simulink model "fwv_2020b"  (R2020b)
settings: Solver=ode15s  StartTime=0.0  StopTime=1  RelTol=1e-3  AbsTol=1e-3  EnableMultiTasking=on
model workspace: external: MATLAB File /home/jeff/文档/research/fwvlab/main.m (data not in the file)
values from neighbouring files (symbols this model uses):
  A_D = 1.5    [main.m]    (also in param.m; params.m)
  A_L = 1.8    [main.m]    (also in param.m; params.m)
  c_bar = S/R    (= 0.0357142857143)    [main.m]    (also in param.m = 0.0251327412287; params.m)
  C_D0 = 0.45    [main.m]    (also in param.m; params.m)
  m = 2    [rbf_pid.m]
  r00 = double(int(f,[0,1]))    [main.m]    (also in param.m = 1; params.m = 0.933333333333)
  r11 = double(int(x*f,[0,1]))    [main.m]    (also in param.m = double(int(curv(x)*(x+1/9),0,1)); params.m = 0.481185185185)
  r22 = double(int(x^2*f,[0,1]))    [main.m]    (also in param.m = double(int(curv(x)*(x+1/9)^2,0,1)); params.m = 0.304750617284)
  r33 = double(int(x^3*f,[0,1]))    [main.m]    (also in param.m = double(int(curv(x)*(x+1/9)^3,0,1)); params.m = 0.218568691358)
  r_cp = Rw*r33/r22    [main.m]    (also in param.m; params.m = 0.10758076225)
  rho = 1.205    [main.m]    (also in param.m; params.m)
  Rw = 0.15    [main.m]    (also in param.m = 0.075; params.m)
  z0 = double(int(f^2,[0,1]))    [main.m]
  z1 = double(int(x*f^2,[0,1]))    [main.m]
  z2 = double(int(x^2*f^2,[0,1]))    [main.m]
undefined symbols (not defined in the file or in its folder): X, Y, Z
libraries: sm_lib x45, nesl_utility x38
(part 2 of 2)

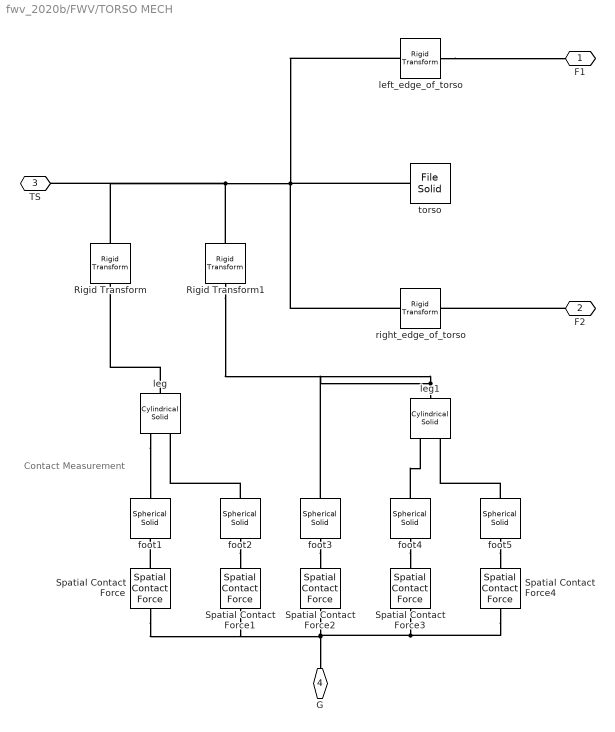
== system fwv_2020b/FWV/TORSO MECH ==
  note: Contact Measurement
  Rigid Transform : sm_lib/Frames and Transforms/Rigid Transform  TranslationMethod=StandardAxis  TranslationStandardOffset=6.25  TranslationLengthUnit=cm  TranslationStandardAxis=-Z  TranslationCartesianOffset=[0 0 0]  TranslationROffset=0  TranslationROffsetUnits=m  TranslationZOffset=0  TranslationZOffsetUnits=m  TranslationThetaOffset=0  TranslationThetaOffsetUnits=deg  RotationMethod=RotationSequence  RotationAngleUnits=deg  RotationStandardAxis=+Y  RotationAngle=90  RotationArbitraryAxis=[0 0 1]  FollAlignAxisA=+X  BaseAlignAxisA=+Y  FollAlignAxisB=+Y  BaseAlignAxisB=+Z  RotationSequenceAxes=FollowerAxes  RotationSequence=ZYX  RotationSequenceAngles=[45 90 0]  RotationSequenceAnglesUnits=deg  RotationMatrix=[1 0 0; 0 1 0; 0 0 1]
  Rigid Transform1 : sm_lib/Frames and Transforms/Rigid Transform  TranslationMethod=StandardAxis  TranslationStandardOffset=6.25  TranslationLengthUnit=cm  TranslationStandardAxis=-Z  TranslationCartesianOffset=[0 0 0]  TranslationROffset=0  TranslationROffsetUnits=m  TranslationZOffset=0  TranslationZOffsetUnits=m  TranslationThetaOffset=0  TranslationThetaOffsetUnits=deg  RotationMethod=RotationSequence  RotationAngleUnits=deg  RotationStandardAxis=+X  RotationAngle=90  RotationArbitraryAxis=[0 0 1]  FollAlignAxisA=+X  BaseAlignAxisA=+Y  FollAlignAxisB=+Y  BaseAlignAxisB=+Z  RotationSequenceAxes=FollowerAxes  RotationSequence=ZYX  RotationSequenceAngles=[-45 90 0]  RotationSequenceAnglesUnits=deg  RotationMatrix=[1 0 0; 0 1 0; 0 0 1]
  Spatial Contact Force{,1..4} (5 alike) : sm_lib/Forces and Torques/Spatial Contact Force  CoefficientOfDynamicFriction=mu1  CoefficientOfStaticFriction=mu0  SenseContactBaseRotation=off  SenseContactBaseTranslation=off  NormalDamping=1e3  NormalDampingUnits=N/(m/s)  SenseContactFollowerRotation=off  SenseContactFollowerTranslation=off  SenseContactSignal=off  NormalStiffness=1e6  NormalStiffnessUnits=N/m  FrictionalCriticalVelocity=1e-3  FrictionalCriticalVelocityUnits=m/s  ZeroCrossDetectContactStartAndEnd=off  FrictionType=SmoothStickSlip  SenseFrictionalForceMagnitude=off  SenseNormalForceMagnitude=off  NormalForceType=SmoothSpringDamper  SenseNormalVelocity=off  SenseSeparationDistance=off  SenseTangentialVelocity=off  SenseTangentialVelocityMagnitude=off  NormalTransitionRegionWidth=1e-4  NormalTransitionRegionWidthUnits=m
  foot{1..5} (5 alike) : sm_lib/Body Elements/Spherical Solid  GraphicAmbientColor=[0.15 0.15 0.15 1.0]  BasedOnType=Density  CenterOfMass=[0 0 0]  CenterOfMassUnits=m  GraphicDiffuseColor=[0.5 0.5 0.5]  Density=1000  DensityUnits=kg/m^3  DoExposeReferenceFrame=on  GraphicEmissiveColor=[0.0 0.0 0.0 1.0]  ExportEntireGeometry=on  SerializedExposedGeometries=<ExposedGeometries><ExposedGeometry><RawGeometryId>entire</RawGeometryId><ExposedGeometryId>G</ExposedGeometryId></ExposedGeometry></ExposedGeometries>  SerializedFrames=<Frames/>  MarkerShape=Sphere  MarkerSize=10  GraphicType=FromGeometry  InertiaType=Custom  Mass=0  MassUnits=kg  MomentsOfInertia=[1 1 1]  MomentsOfInertiaUnits=kg*m^2  GraphicOpacity=1.0  ProductsOfInertia=[0 0 0]  ProductsOfInertiaUnits=kg*m^2  GraphicShininess=75  GraphicSpecularColor=[0.5 0.5 0.5 1.0]  SphereRadius=0.25  SphereRadiusUnits=cm  GraphicVisPropType=SimpleVisualProperties
  left_edge_of_torso : sm_lib/Frames and Transforms/Rigid Transform  TranslationMethod=Cartesian  TranslationStandardOffset=0  TranslationLengthUnit=cm  TranslationStandardAxis=+Z  TranslationCartesianOffset=[0 4 0]  TranslationROffset=0  TranslationROffsetUnits=m  TranslationZOffset=0  TranslationZOffsetUnits=m  TranslationThetaOffset=0  TranslationThetaOffsetUnits=deg  RotationMethod=None  RotationAngleUnits=deg  RotationStandardAxis=+Z  RotationAngle=0.0  RotationArbitraryAxis=[0 0 1]  FollAlignAxisA=+X  BaseAlignAxisA=+Y  FollAlignAxisB=+Y  BaseAlignAxisB=+Z  RotationSequenceAxes=FollowerAxes  RotationSequence=XYX  RotationSequenceAngles=[0 0 0]  RotationSequenceAnglesUnits=deg  RotationMatrix=[1 0 0; 0 1 0; 0 0 1]
  leg : sm_lib/Body Elements/Cylindrical Solid  GraphicAmbientColor=[0.15 0.15 0.15 1.0]  BasedOnType=Density  CenterOfMass=[0 0 0]  CenterOfMassUnits=m  GraphicDiffuseColor=[0.5 0.5 0.5]  CylinderLength=160  CylinderLengthUnits=mm  CylinderRadius=2.5  CylinderRadiusUnits=mm  Density=1000  DensityUnits=kg/m^3  DoExposeReferenceFrame=on  GraphicEmissiveColor=[0.0 0.0 0.0 1.0]  ExportEntireGeometry=off  SerializedFrames=<Frames><Frame><Id>Frame1</Id><Value><Name>F1</Name><Origin><Source>GeometricFeature</Source><FeatureName>top curve</FeatureName></Origin><PrimaryAxis><DefinedDirection>+Z</DefinedDirection><Source>ReferenceFrame</Source><SourceDirection>+Z</SourceDirection><FeatureName></FeatureName></PrimaryAxis><SecondaryAxis><DefinedDirection>+X</DefinedDirection><Source>ReferenceFrame</Source><SourceDirection>+X</SourceDirection><FeatureName></FeatureName></SecondaryAxis></Value></Frame><Frame><Id>Frame2</Id><Value><Name>F2</Name><Origin><Source>GeometricFeature</Source><FeatureName>bottom curve</FeatureName></Origin><PrimaryAxis><DefinedDirection>-Z</DefinedDirection><Source>ReferenceFrame</Source><SourceDirection>+Z</SourceDirection><FeatureName></FeatureName></PrimaryAxis><SecondaryAxis><DefinedDirection>+X</DefinedDirection><Source>ReferenceFrame</Source><SourceDirection>+X</SourceDirection><FeatureName></FeatureName></SecondaryAxis></Value></Frame></Frames>  MarkerShape=Sphere  MarkerSize=10  GraphicType=FromGeometry  InertiaType=CalculateFromGeometry  Mass=1  MassUnits=kg  MomentsOfInertia=[1 1 1]  MomentsOfInertiaUnits=kg*m^2  GraphicOpacity=1.0  ProductsOfInertia=[0 0 0]  ProductsOfInertiaUnits=kg*m^2  GraphicShininess=75  GraphicSpecularColor=[0.5 0.5 0.5 1.0]  GraphicVisPropType=SimpleVisualProperties
  leg1 : sm_lib/Body Elements/Cylindrical Solid  GraphicAmbientColor=[0.15 0.15 0.15 1.0]  BasedOnType=Density  CenterOfMass=[0 0 0]  CenterOfMassUnits=m  GraphicDiffuseColor=[0.5 0.5 0.5]  CylinderLength=160  CylinderLengthUnits=mm  CylinderRadius=2.5  CylinderRadiusUnits=mm  Density=800  DensityUnits=kg/m^3  DoExposeReferenceFrame=on  GraphicEmissiveColor=[0.0 0.0 0.0 1.0]  ExportEntireGeometry=off  SerializedFrames=<Frames><Frame><Id>Frame1</Id><Value><Name>F1</Name><Origin><Source>GeometricFeature</Source><FeatureName>top curve</FeatureName></Origin><PrimaryAxis><DefinedDirection>+Z</DefinedDirection><Source>ReferenceFrame</Source><SourceDirection>+Z</SourceDirection><FeatureName></FeatureName></PrimaryAxis><SecondaryAxis><DefinedDirection>+X</DefinedDirection><Source>ReferenceFrame</Source><SourceDirection>+X</SourceDirection><FeatureName></FeatureName></SecondaryAxis></Value></Frame><Frame><Id>Frame2</Id><Value><Name>F2</Name><Origin><Source>GeometricFeature</Source><FeatureName>bottom curve</FeatureName></Origin><PrimaryAxis><DefinedDirection>-Z</DefinedDirection><Source>ReferenceFrame</Source><SourceDirection>+Z</SourceDirection><FeatureName></FeatureName></PrimaryAxis><SecondaryAxis><DefinedDirection>+X</DefinedDirection><Source>ReferenceFrame</Source><SourceDirection>+X</SourceDirection><FeatureName></FeatureName></SecondaryAxis></Value></Frame></Frames>  MarkerShape=Sphere  MarkerSize=10  GraphicType=FromGeometry  InertiaType=CalculateFromGeometry  Mass=1  MassUnits=kg  MomentsOfInertia=[1 1 1]  MomentsOfInertiaUnits=kg*m^2  GraphicOpacity=1.0  ProductsOfInertia=[0 0 0]  ProductsOfInertiaUnits=kg*m^2  GraphicShininess=75  GraphicSpecularColor=[0.5 0.5 0.5 1.0]  GraphicVisPropType=SimpleVisualProperties
  right_edge_of_torso : sm_lib/Frames and Transforms/Rigid Transform  TranslationMethod=Cartesian  TranslationStandardOffset=0  TranslationLengthUnit=cm  TranslationStandardAxis=+Z  TranslationCartesianOffset=[0 -4 0]  TranslationROffset=0  TranslationROffsetUnits=m  TranslationZOffset=0  TranslationZOffsetUnits=m  TranslationThetaOffset=0  TranslationThetaOffsetUnits=deg  RotationMethod=StandardAxis  RotationAngleUnits=deg  RotationStandardAxis=+X  RotationAngle=180  RotationArbitraryAxis=[0 0 1]  FollAlignAxisA=+X  BaseAlignAxisA=+Y  FollAlignAxisB=+Y  BaseAlignAxisB=+Z  RotationSequenceAxes=FollowerAxes  RotationSequence=XYX  RotationSequenceAngles=[0 0 0]  RotationSequenceAnglesUnits=deg  RotationMatrix=[1 0 0; 0 1 0; 0 0 1]
  torso : sm_lib/Body Elements/File Solid  ExtGeomFileName=meshes/body.step  UnitType=FromFile  ExtGeomFileUnits=m  StepReaderType=HEX  ExportConvexHullGeometry=off  InertiaType=CalculateFromGeometry  Mass=30  MassUnits=g  CenterOfMass=[0 0 0]  CenterOfMassUnits=m  MomentsOfInertia=[1 1 1]  MomentsOfInertiaUnits=kg*m^2  ProductsOfInertia=[0 0 0]  ProductsOfInertiaUnits=kg*m^2  BasedOnType=Mass  Density=1000  DensityUnits=kg/m^3  DoExposeReferenceFrame=on  SerializedFrames=<Frames/>  GraphicType=FromGeometry  MarkerShape=Sphere  MarkerSize=10  GraphicVisPropType=SimpleVisualProperties  GraphicDiffuseColor=[0.5 0.5 0.5]  GraphicSpecularColor=[0.5 0.5 0.5 1.0]  GraphicAmbientColor=[0.15 0.15 0.15 1.0]  GraphicEmissiveColor=[0.0 0.0 0.0 1.0]  GraphicShininess=75  GraphicOpacity=1.0
  F1 : PMIOPort  Side=Right
  F2 : PMIOPort  Port=2  Side=Left
  TS : PMIOPort  Port=3  Side=Left
  G : PMIOPort  Port=4  Side=Right
  connections:
  Spatial Contact Force3/LConn1 -- Spatial Contact Force/LConn1 -- Spatial Contact Force1/LConn1 -- G/RConn1 -- Spatial Contact Force2/LConn1 -- Spatial Contact Force4/LConn1
  Rigid Transform1/LConn1 -- right_edge_of_torso/LConn1 -- torso/RConn1 -- left_edge_of_torso/LConn1 -- Rigid Transform/LConn1 -- TS/RConn1
  leg1/RConn1 -- Rigid Transform1/RConn1 -- foot3/RConn1
  leg/LConn1 -- foot1/RConn1
  Spatial Contact Force/RConn1 -- foot1/LConn1
  foot2/LConn1 -- Spatial Contact Force1/RConn1
  left_edge_of_torso/RConn1 -- F1/RConn1
  foot2/RConn1 -- leg/LConn2
  foot5/LConn1 -- Spatial Contact Force4/RConn1
  leg/RConn1 -- Rigid Transform/RConn1
  F2/RConn1 -- right_edge_of_torso/RConn1
  foot4/RConn1 -- leg1/LConn1
  foot5/RConn1 -- leg1/LConn2
  foot3/LConn1 -- Spatial Contact Force2/RConn1
  foot4/LConn1 -- Spatial Contact Force3/RConn1

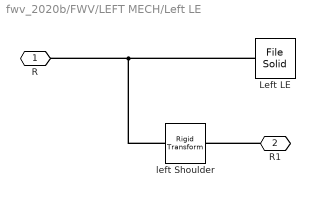
== system fwv_2020b/FWV/LEFT MECH/Left LE ==
  Left LE : sm_lib/Body Elements/File Solid  ExtGeomFileName=meshes/left_LE.step  UnitType=FromFile  ExtGeomFileUnits=m  StepReaderType=HEX  ExportConvexHullGeometry=off  InertiaType=CalculateFromGeometry  Mass=1  MassUnits=kg  CenterOfMass=[0 0 0]  CenterOfMassUnits=m  MomentsOfInertia=[1 1 1]  MomentsOfInertiaUnits=kg*m^2  ProductsOfInertia=[0 0 0]  ProductsOfInertiaUnits=kg*m^2  BasedOnType=Density  Density=800  DensityUnits=kg/m^3  DoExposeReferenceFrame=on  SerializedFrames=<Frames/>  GraphicType=FromGeometry  MarkerShape=Sphere  MarkerSize=10  GraphicVisPropType=SimpleVisualProperties  GraphicDiffuseColor=[0.5 0.5 0.5]  GraphicSpecularColor=[0.5 0.5 0.5 1.0]  GraphicAmbientColor=[0.15 0.15 0.15 1.0]  GraphicEmissiveColor=[0.0 0.0 0.0 1.0]  GraphicShininess=75  GraphicOpacity=1.0
  left Shoulder : sm_lib/Frames and Transforms/Rigid Transform  TranslationMethod=Cartesian  TranslationStandardOffset=0  TranslationLengthUnit=cm  TranslationStandardAxis=+Z  TranslationCartesianOffset=[0 1 4]  TranslationROffset=0  TranslationROffsetUnits=m  TranslationZOffset=0  TranslationZOffsetUnits=m  TranslationThetaOffset=0  TranslationThetaOffsetUnits=deg  RotationMethod=StandardAxis  RotationAngleUnits=deg  RotationStandardAxis=+X  RotationAngle=-90  RotationArbitraryAxis=[0 0 1]  FollAlignAxisA=+X  BaseAlignAxisA=+Y  FollAlignAxisB=+Y  BaseAlignAxisB=+Z  RotationSequenceAxes=FollowerAxes  RotationSequence=XYX  RotationSequenceAngles=[0 0 0]  RotationSequenceAnglesUnits=deg  RotationMatrix=[0 1 0; 0 0 1; 1 0 0]
  R : PMIOPort  Side=Left
  R1 : PMIOPort  Port=2  Side=Right
  connections:
  R1/RConn1 -- left Shoulder/RConn1
  Left LE/RConn1 -- left Shoulder/LConn1 -- R/RConn1

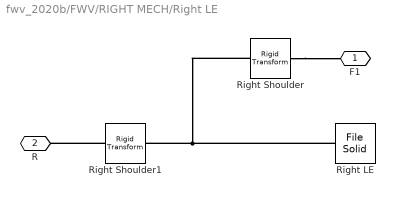
== system fwv_2020b/FWV/RIGHT MECH/Right LE ==
  Right LE : sm_lib/Body Elements/File Solid  ExtGeomFileName=meshes/right_LE.step  UnitType=FromFile  ExtGeomFileUnits=m  StepReaderType=HEX  ExportConvexHullGeometry=off  InertiaType=CalculateFromGeometry  Mass=1  MassUnits=kg  CenterOfMass=[0 0 0]  CenterOfMassUnits=m  MomentsOfInertia=[1 1 1]  MomentsOfInertiaUnits=kg*m^2  ProductsOfInertia=[0 0 0]  ProductsOfInertiaUnits=kg*m^2  BasedOnType=Density  Density=800  DensityUnits=kg/m^3  DoExposeReferenceFrame=on  SerializedFrames=<Frames/>  GraphicType=FromGeometry  MarkerShape=Sphere  MarkerSize=10  GraphicVisPropType=SimpleVisualProperties  GraphicDiffuseColor=[0.5 0.5 0.5]  GraphicSpecularColor=[0.5 0.5 0.5 1.0]  GraphicAmbientColor=[0.15 0.15 0.15 1.0]  GraphicEmissiveColor=[0.0 0.0 0.0 1.0]  GraphicShininess=75  GraphicOpacity=1.0
  Right Shoulder : sm_lib/Frames and Transforms/Rigid Transform  TranslationMethod=Cartesian  TranslationStandardOffset=0  TranslationLengthUnit=cm  TranslationStandardAxis=+Z  TranslationCartesianOffset=[0 -1 4]  TranslationROffset=0  TranslationROffsetUnits=m  TranslationZOffset=0  TranslationZOffsetUnits=m  TranslationThetaOffset=0  TranslationThetaOffsetUnits=deg  RotationMethod=StandardAxis  RotationAngleUnits=deg  RotationStandardAxis=+X  RotationAngle=-90  RotationArbitraryAxis=[0 0 1]  FollAlignAxisA=+X  BaseAlignAxisA=+Y  FollAlignAxisB=+Y  BaseAlignAxisB=+Z  RotationSequenceAxes=FollowerAxes  RotationSequence=XYX  RotationSequenceAngles=[0 0 0]  RotationSequenceAnglesUnits=deg  RotationMatrix=[0 1 0; 0 0 1; 1 0 0]
  Right Shoulder1 : sm_lib/Frames and Transforms/Rigid Transform  TranslationMethod=None  TranslationStandardOffset=0  TranslationLengthUnit=cm  TranslationStandardAxis=+Z  TranslationCartesianOffset=[0 -1 4]  TranslationROffset=0  TranslationROffsetUnits=m  TranslationZOffset=0  TranslationZOffsetUnits=m  TranslationThetaOffset=0  TranslationThetaOffsetUnits=deg  RotationMethod=StandardAxis  RotationAngleUnits=deg  RotationStandardAxis=+X  RotationAngle=180  RotationArbitraryAxis=[0 0 1]  FollAlignAxisA=+X  BaseAlignAxisA=+Y  FollAlignAxisB=+Y  BaseAlignAxisB=+Z  RotationSequenceAxes=FollowerAxes  RotationSequence=XYX  RotationSequenceAngles=[0 0 0]  RotationSequenceAnglesUnits=deg  RotationMatrix=[0 1 0; 0 0 1; 1 0 0]
  F1 : PMIOPort  Side=Right
  R : PMIOPort  Port=2  Side=Left
  connections:
  Right Shoulder/LConn1 -- Right LE/RConn1 -- Right Shoulder1/RConn1
  Right Shoulder/RConn1 -- F1/RConn1
  Right Shoulder1/LConn1 -- R/RConn1

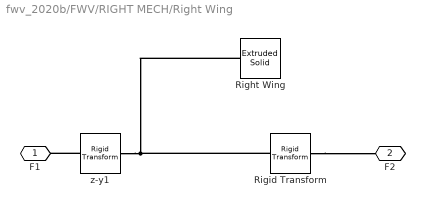
== system fwv_2020b/FWV/RIGHT MECH/Right Wing ==
  Right Wing : sm_lib/Body Elements/Extruded Solid  GraphicAmbientColor=[0.15 0.15 0.15 1.0]  BasedOnType=Density  CenterOfMass=[0 0 0]  CenterOfMassUnits=m  GraphicDiffuseColor=[0.5 0.5 0.5]  ExportConvexHullGeometry=off  ExtrusionCrossSection=[0 0; -140 0; -140 -25; -20 -50]  ExtrusionCrossSectionUnits=mm  Density=rho_w  DensityUnits=kg/m^3  DoExposeReferenceFrame=off  GraphicEmissiveColor=[0.0 0.0 0.0 1.0]  ExportEntireGeometry=off  ExtrusionLength=0.06  ExtrusionLengthUnits=mm  ExtrusionType=General  SerializedFrames=<Frames><Frame><Id>Frame1</Id><Value><Name>F1</Name><Origin><Source>ReferenceFrame</Source><FeatureName></FeatureName></Origin><PrimaryAxis><DefinedDirection>+X</DefinedDirection><Source>ReferenceFrame</Source><SourceDirection>+Z</SourceDirection><FeatureName></FeatureName></PrimaryAxis><SecondaryAxis><DefinedDirection>+Y</DefinedDirection><Source>ReferenceFrame</Source><SourceDirection>+X</SourceDirection><FeatureName></FeatureName></SecondaryAxis></Value></Frame></Frames>  MarkerShape=Sphere  MarkerSize=10  GraphicType=FromGeometry  InertiaType=CalculateFromGeometry  Mass=1  MassUnits=kg  MomentsOfInertia=[1 1 1]  MomentsOfInertiaUnits=kg*m^2  PolygonNumSides=3  GraphicOpacity=1.0  PolygonOuterRadius=1  PolygonOuterRadiusUnits=m  ProductsOfInertia=[0 0 0]  ProductsOfInertiaUnits=kg*m^2  GraphicShininess=75  GraphicSpecularColor=[0.5 0.5 0.5 1.0]  GraphicVisPropType=SimpleVisualProperties
  Rigid Transform : sm_lib/Frames and Transforms/Rigid Transform  TranslationMethod=Cartesian  TranslationStandardOffset=r_cp  TranslationLengthUnit=m  TranslationStandardAxis=-Y  TranslationCartesianOffset=[0 -r_cp 0]  TranslationROffset=0  TranslationROffsetUnits=m  TranslationZOffset=0  TranslationZOffsetUnits=m  TranslationThetaOffset=0  TranslationThetaOffsetUnits=deg  RotationMethod=None  RotationAngleUnits=deg  RotationStandardAxis=+Z  RotationAngle=0.0  RotationArbitraryAxis=[0 0 1]  FollAlignAxisA=+X  BaseAlignAxisA=+Y  FollAlignAxisB=+Y  BaseAlignAxisB=+Z  RotationSequenceAxes=FollowerAxes  RotationSequence=XYX  RotationSequenceAngles=[0 0 0]  RotationSequenceAnglesUnits=deg  RotationMatrix=[1 0 0; 0 1 0; 0 0 1]
  z-y1 : sm_lib/Frames and Transforms/Rigid Transform  TranslationMethod=None  TranslationStandardOffset=0  TranslationLengthUnit=cm  TranslationStandardAxis=+Z  TranslationCartesianOffset=[0 1 4]  TranslationROffset=0  TranslationROffsetUnits=m  TranslationZOffset=0  TranslationZOffsetUnits=m  TranslationThetaOffset=0  TranslationThetaOffsetUnits=deg  RotationMethod=StandardAxis  RotationAngleUnits=deg  RotationStandardAxis=+X  RotationAngle=90  RotationArbitraryAxis=[0 0 1]  FollAlignAxisA=+X  BaseAlignAxisA=+Y  FollAlignAxisB=+Y  BaseAlignAxisB=+Z  RotationSequenceAxes=FollowerAxes  RotationSequence=XYX  RotationSequenceAngles=[0 0 0]  RotationSequenceAnglesUnits=deg  RotationMatrix=[0 0 1; 1 0 0; 0 1 0]
  F1 : PMIOPort  Side=Left
  F2 : PMIOPort  Port=2  Side=Right
  connections:
  Rigid Transform/RConn1 -- F2/RConn1
  Rigid Transform/LConn1 -- Right Wing/LConn1 -- z-y1/RConn1
  z-y1/LConn1 -- F1/RConn1

== matlab function fwv_2020b/AeroDynamic/aero force and moment ==
  data: le0 input; F_N output; alpha input; M_rd output; d_cp output; rot_dot input; A_L parameter; A_D parameter; C_D0 parameter; rho parameter; c_bar parameter; Rw parameter; r22 parameter; r11 parameter; r00 parameter; z2 parameter; z1 parameter; z0 parameter
function [F_N,M_rd,d_cp] = fcn(le0, alpha, rot_dot, A_L, A_D, C_D0, rho, c_bar, Rw, r22, r11, r00, z2, z1, z0)
a2=le0(3)^2+le0(4)^2;
a1=2*(le0(1)*le0(3)+le0(2)*le0(4));
a0=le0(1)^2+le0(2)^2;
C_L=A_L*sin(2*alpha);
C_D=C_D0+A_D*(1-cos(2*alpha));
C_N=C_L*cos(alpha)+C_D*sin(alpha);
F_N=-0.5*rho*C_N*c_bar*(a2*Rw^3*r22+a1*Rw^2*r11+a0*Rw*r00);
d_cp_=0.82/pi*(mod(abs(alpha),pi))+0.05;
M_ae=-0.5*rho*C_N*c_bar^2*d_cp_*(a2*Rw^3*z2+a1*Rw^2*z1+a0*Rw*z0);
if F_N==0
d_cp=-0.51*c_bar;
else
    d_cp=-M_ae/F_N;
end
M_rd=0;

== matlab function fwv_2020b/AeroDynamic/AoA ==
  data: le0 input; alpha output; rot input; Rw parameter; r33 parameter; r22 parameter
function alpha = fcn(le0, rot, Rw, r33, r22)
rcp = Rw*r33/r22;
vi = le0(1)+le0(3)*rcp;
vo = le0(2)+le0(4)*rcp;
dir_v = atan2(vo,vi);
if vi~=0
    alpha = -rot + sign(vi)*pi/2 - atan(vo/vi);
else
    alpha = 0;
end

== matlab function fwv_2020b/AeroDynamic/LE root vel ==
  data: vt input; le0 output; wt input; stk input; wstk input
function le0 = fcn(vt, wt, stk, wstk)
% vt and wt refer to the vel of torso. vs and ws refer to the vel of
% shoulder. vl and wl refer to the vel of leading edge. We pick out the
% index x & z for further usage. stk and wstk are stroke meaning.
d0=0.05;
ds=0.04;
rts = [0 d0 ds];
vs = vt + cross(wt,rts);
ws = wt;
C_stk = cos(stk);
S_stk = sin(stk);
vl = [C_stk * vs(1) + S_stk * vs(2), -S_stk * vs(1) + C_stk*vs(2), vs(3)];
wl = [C_stk * ws(1) + S_stk * ws(2), -S_stk * ws(1) + C_stk*ws(2), ws(3) + wstk];
le0 = [vl(1),-wl(3);vl(3),wl(1)];

== matlab function fwv_2020b/AeroDynamic/world to body frame ==
  data: q input; vb output; v input; w input; wb output
function [vb,wb] = world2body(q,v,w)
S1 = sin(q(1)); C1 = cos(q(1)); S2 = sin(q(2)); C2 = cos(q(2));
S3 = sin(q(3)); C3 = cos(q(3));
vb = [C2*C3*v(1)+C2*S3*v(2)-S2*v(3),(S1*S2*C3-S1*S3)*v(1)+(S1*S2*S3+S1*S3)*v(2)+S1*C2*v(3),(C1*S2*C3+S1*S3)*v(1)+(C1*S2*S3-S1*C3)*v(2)+C1*C2*v(3)];
wb = [w(1)-S2*w(3), C1*w(2)+C2*S1*w(3), -S1*w(2)+C2*C1*w(3)];

== matlab function fwv_2020b/AeroDynamic/LE root vel1 ==
  data: vt input; le0 output; wt input; stk input; wstk input
function le0 = fcn(vt, wt, stk, wstk)
% vt and wt refer to the vel of torso. vs and ws refer to the vel of
% shoulder. vl and wl refer to the vel of leading edge. We pick out the
% index x & z for further usage. stk and wstk are stroke meaning.
d0=-0.05;
ds=0.04;
rts = [0 d0 ds];
vs = vt + cross(wt,rts);
ws = wt;
C_stk = cos(-stk);
S_stk = sin(-stk);
vl = [C_stk * vs(1) + S_stk * vs(2), -S_stk * vs(1) + C_stk*vs(2), vs(3)];
wl = [C_stk * ws(1) + S_stk * ws(2), -S_stk * ws(1) + C_stk*ws(2), ws(3) - wstk];
le0 = [vl(1),-wl(3);vl(3),wl(1)];

== matlab function fwv_2020b/AeroDynamic/AoA1 ==
  data: le0 input; alpha output; rot input; Rw parameter; r33 parameter; r22 parameter
function alpha = fcn(le0, rot, Rw, r33, r22)
rcp = -Rw*r33/r22;
vi = le0(1)+le0(3)*rcp;
vo = le0(2)+le0(4)*rcp;
if vi~=0
    alpha = -rot + sign(vi)*pi/2 - atan(vo/vi);
else
    alpha = 0;
end

== matlab function fwv_2020b/AeroDynamic/aero force and moment1 ==
  data: le0 input; F_N output; alpha input; M_rd output; d_cp output; rot_dot input; A_L parameter; A_D parameter; C_D0 parameter; rho parameter; c_bar parameter; Rw parameter; r22 parameter; r11 parameter; r00 parameter; z2 parameter; z1 parameter; z0 parameter
function [F_N,M_rd,d_cp] = fcn(le0, alpha, rot_dot, A_L, A_D, C_D0, rho, c_bar, Rw, r22, r11, r00, z2, z1, z0)
a2=le0(3)^2+le0(4)^2;
a1=-2*(le0(1)*le0(3)+le0(2)*le0(4));
a0=le0(1)^2+le0(2)^2;
C_L=A_L*sin(2*alpha);
C_D=C_D0+A_D*(1-cos(2*alpha));
C_N=C_L*cos(alpha)+C_D*sin(alpha);
F_N=-0.5*rho*C_N*c_bar*(a2*Rw^3*r22+a1*Rw^2*r11+a0*Rw*r00);
d_cp_=0.82/pi*(mod(abs(alpha),pi))+0.05;
M_ae=-0.5*rho*C_N*c_bar^2*d_cp_*(a2*Rw^3*z2+a1*Rw^2*z1+a0*Rw*z0);
if F_N==0
d_cp=-0.51*c_bar;
else
    d_cp=-M_ae/F_N;
end
M_rd=0;
